simulink model "Simulink_model_pre_alpha"  (R2022b)
settings: Solver=VariableStepAuto  StartTime=0.0  StopTime=10.0  RelTol=1e-3
settings Model: Creator=user  LastModifiedBy=user

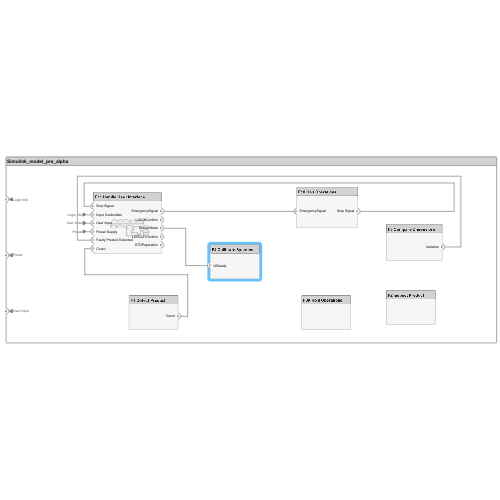
[thumbnail: Simulink's stored preview of the top-level diagram]
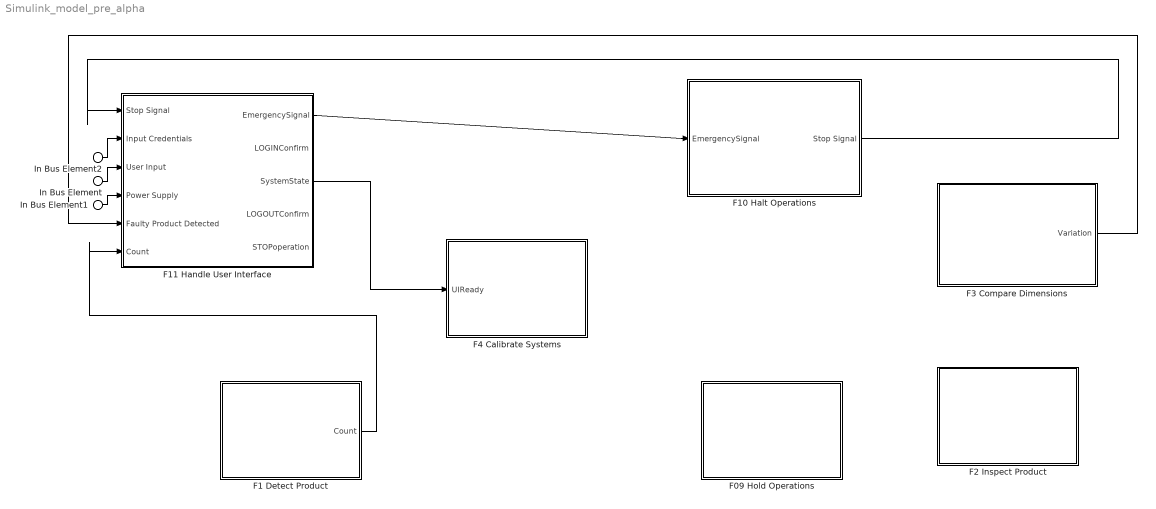
== system Simulink_model_pre_alpha ==
  In Bus Element2 : Inport  PortName=Login info
  In Bus Element1 : Inport  Port=2  PortName=Power
  In Bus Element : Inport  Port=3  PortName=User Input
  F09 Hold Operations : Subsystem
      settings: PortSchema="{\"entries\":[{\"content\":{\"headerSize\":26,\"margin\":15,\"minimumSpacing\":25,\"sides\":[{\"content\":{\"connectorIds\":[]},\"type\":\"ConnectorPlacement.EquallySpacedRectSide\",\"uuid\":\"0eb90d47-70e1-4803-9acf-c665eca2c33b\"},{\"content\":{\"connectorIds\":[],\"side\":\"RIGHT\"},\"type\":\"ConnectorPlacement.EquallySpacedRectSide\",\"uuid\":\"4ca2a7b5-05ae-49c5-bdeb-54cebcfbfa14\"},{\"content\":{\"connectorIds\":[],\"side\":\"TOP\"},\"type\":\"ConnectorPlacement.EquallySpacedRectSide\",\"uuid\":\"0ca0afdf-f9df-4611-9068-250b443486a2\"}]},\"type\":\"ConnectorPlacement.EquallySpacedConnector\",\"uuid\":\"958f48af-2ef9-4d0f-b00d-a4686f354a93\"}],\"packageUris\":[\"http://schema.mathworks.com/mf0/Connector/R2020b\"],\"version\":\"1.0\"}"
  F1 Detect Product : Subsystem
      settings: PortSchema="{\"entries\":[{\"content\":{\"headerSize\":26,\"margin\":15,\"minimumSpacing\":25,\"sides\":[{\"content\":{\"connectorIds\":[]},\"type\":\"ConnectorPlacement.EquallySpacedRectSide\",\"uuid\":\"0eb90d47-70e1-4803-9acf-c665eca2c33b\"},{\"content\":{\"connectorIds\":[\"Out1\"],\"side\":\"RIGHT\"},\"type\":\"ConnectorPlacement.EquallySpacedRectSide\",\"uuid\":\"4ca2a7b5-05ae-49c5-bdeb-54cebcfbfa14\"},{\"content\":{\"connectorIds\":[],\"side\":\"TOP\"},\"type\":\"ConnectorPlacement.EquallySpacedRectSide\",\"uuid\":\"0ca0afdf-f9df-4611-9068-250b443486a2\"}]},\"type\":\"ConnectorPlacement.EquallySpacedConnector\",\"uuid\":\"958f48af-2ef9-4d0f-b00d-a4686f354a93\"}],\"packageUris\":[\"http://schema.mathworks.com/mf0/Connector/R2020b\"],\"version\":\"1.0\"}"
  F10 Halt Operations : Subsystem
      settings: PortSchema="{\"entries\":[{\"content\":{\"headerSize\":26,\"margin\":15,\"minimumSpacing\":25,\"sides\":[{\"content\":{\"connectorIds\":[\"In1\"]},\"type\":\"ConnectorPlacement.EquallySpacedRectSide\",\"uuid\":\"0eb90d47-70e1-4803-9acf-c665eca2c33b\"},{\"content\":{\"connectorIds\":[\"Out1\"],\"side\":\"RIGHT\"},\"type\":\"ConnectorPlacement.EquallySpacedRectSide\",\"uuid\":\"4ca2a7b5-05ae-49c5-bdeb-54cebcfbfa14\"},{\"content\":{\"connectorIds\":[],\"side\":\"TOP\"},\"type\":\"ConnectorPlacement.EquallySpacedRectSide\",\"uuid\":\"0ca0afdf-f9df-4611-9068-250b443486a2\"}]},\"type\":\"ConnectorPlacement.EquallySpacedConnector\",\"uuid\":\"958f48af-2ef9-4d0f-b00d-a4686f354a93\"}],\"packageUris\":[\"http://schema.mathworks.com/mf0/Connector/R2020b\"],\"version\":\"1.0\"}"
  F11 Handle User Interface : Subsystem
      settings: PortSchema="{\"entries\":[{\"content\":{\"headerSize\":26,\"margin\":15,\"minimumSpacing\":25,\"sides\":[{\"content\":{\"connectorIds\":[\"In1\",\"In2\",\"In3\",\"In4\",\"In5\",\"In6\"]},\"type\":\"ConnectorPlacement.EquallySpacedRectSide\",\"uuid\":\"0eb90d47-70e1-4803-9acf-c665eca2c33b\"},{\"content\":{\"connectorIds\":[\"Out1\",\"Out2\",\"Out3\",\"Out4\",\"Out5\"],\"side\":\"RIGHT\"},\"type\":\"ConnectorPlacement.EquallySpacedRectSide\",\"uuid\":\"4ca2a7b5-05ae-49c5-bdeb-54cebcfbfa14\"},{\"content\":{\"connectorIds\":[],\"side\":\"TOP\"},\"type\":\"ConnectorPlacement.EquallySpacedRectSide\",\"uuid\":\"0ca0afdf-f9df-4611-9068-250b443486a2\"}]},\"type\":\"ConnectorPlacement.EquallySpacedConnector\",\"uuid\":\"958f48af-2ef9-4d0f-b00d-a4686f354a93\"}],\"packageUris\":[\"http://schema.mathworks.com/mf0/Connector/R2020b\"],\"version\":\"1.0\"}"
  F2 Inspect Product : Subsystem
      settings: PortSchema="{\"entries\":[{\"content\":{\"headerSize\":26,\"margin\":15,\"minimumSpacing\":25,\"sides\":[{\"content\":{\"connectorIds\":[]},\"type\":\"ConnectorPlacement.EquallySpacedRectSide\",\"uuid\":\"0eb90d47-70e1-4803-9acf-c665eca2c33b\"},{\"content\":{\"connectorIds\":[],\"side\":\"RIGHT\"},\"type\":\"ConnectorPlacement.EquallySpacedRectSide\",\"uuid\":\"4ca2a7b5-05ae-49c5-bdeb-54cebcfbfa14\"},{\"content\":{\"connectorIds\":[],\"side\":\"TOP\"},\"type\":\"ConnectorPlacement.EquallySpacedRectSide\",\"uuid\":\"0ca0afdf-f9df-4611-9068-250b443486a2\"}]},\"type\":\"ConnectorPlacement.EquallySpacedConnector\",\"uuid\":\"958f48af-2ef9-4d0f-b00d-a4686f354a93\"}],\"packageUris\":[\"http://schema.mathworks.com/mf0/Connector/R2020b\"],\"version\":\"1.0\"}"
  F3 Compare Dimensions : Subsystem
      settings: PortSchema="{\"entries\":[{\"content\":{\"headerSize\":26,\"margin\":15,\"minimumSpacing\":25,\"sides\":[{\"content\":{\"connectorIds\":[]},\"type\":\"ConnectorPlacement.EquallySpacedRectSide\",\"uuid\":\"0eb90d47-70e1-4803-9acf-c665eca2c33b\"},{\"content\":{\"connectorIds\":[\"Out1\"],\"side\":\"RIGHT\"},\"type\":\"ConnectorPlacement.EquallySpacedRectSide\",\"uuid\":\"4ca2a7b5-05ae-49c5-bdeb-54cebcfbfa14\"},{\"content\":{\"connectorIds\":[],\"side\":\"TOP\"},\"type\":\"ConnectorPlacement.EquallySpacedRectSide\",\"uuid\":\"0ca0afdf-f9df-4611-9068-250b443486a2\"}]},\"type\":\"ConnectorPlacement.EquallySpacedConnector\",\"uuid\":\"958f48af-2ef9-4d0f-b00d-a4686f354a93\"}],\"packageUris\":[\"http://schema.mathworks.com/mf0/Connector/R2020b\"],\"version\":\"1.0\"}"
  "F4 Calibrate Systems " : Subsystem
      settings: PortSchema="{\"entries\":[{\"content\":{\"headerSize\":26,\"margin\":15,\"minimumSpacing\":25,\"sides\":[{\"content\":{\"connectorIds\":[\"In1\"]},\"type\":\"ConnectorPlacement.EquallySpacedRectSide\",\"uuid\":\"0eb90d47-70e1-4803-9acf-c665eca2c33b\"},{\"content\":{\"connectorIds\":[],\"side\":\"RIGHT\"},\"type\":\"ConnectorPlacement.EquallySpacedRectSide\",\"uuid\":\"4ca2a7b5-05ae-49c5-bdeb-54cebcfbfa14\"},{\"content\":{\"connectorIds\":[],\"side\":\"TOP\"},\"type\":\"ConnectorPlacement.EquallySpacedRectSide\",\"uuid\":\"0ca0afdf-f9df-4611-9068-250b443486a2\"}]},\"type\":\"ConnectorPlacement.EquallySpacedConnector\",\"uuid\":\"958f48af-2ef9-4d0f-b00d-a4686f354a93\"}],\"packageUris\":[\"http://schema.mathworks.com/mf0/Connector/R2020b\"],\"version\":\"1.0\"}"
  wires:
  In Bus Element1/1 -> F11 Handle User Interface/4(Power Supply)
  F10 Halt Operations/1(Stop Signal) -> F11 Handle User Interface/1(Stop Signal)
  In Bus Element/1 -> F11 Handle User Interface/3(User Input)
  In Bus Element2/1 -> F11 Handle User Interface/2(Input Credentials)
  F3 Compare Dimensions/1(Variation) -> F11 Handle User Interface/5(Faulty Product Detected)
  F1 Detect Product/1(Count) -> F11 Handle User Interface/6(Count)
  F11 Handle User Interface/3(SystemState) -> "F4 Calibrate Systems "/1(UIReady)
  F11 Handle User Interface/1(EmergencySignal) -> F10 Halt Operations/1(EmergencySignal)

== system Simulink_model_pre_alpha/F09 Hold Operations ==

== system Simulink_model_pre_alpha/F1 Detect Product ==
  Bus Element Out1 : Outport  PortName=Count

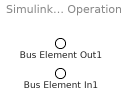
== system Simulink_model_pre_alpha/F10 Halt Operations ==
  Bus Element In1 : Inport  PortName=EmergencySignal
  Bus Element Out1 : Outport  PortName=Stop Signal

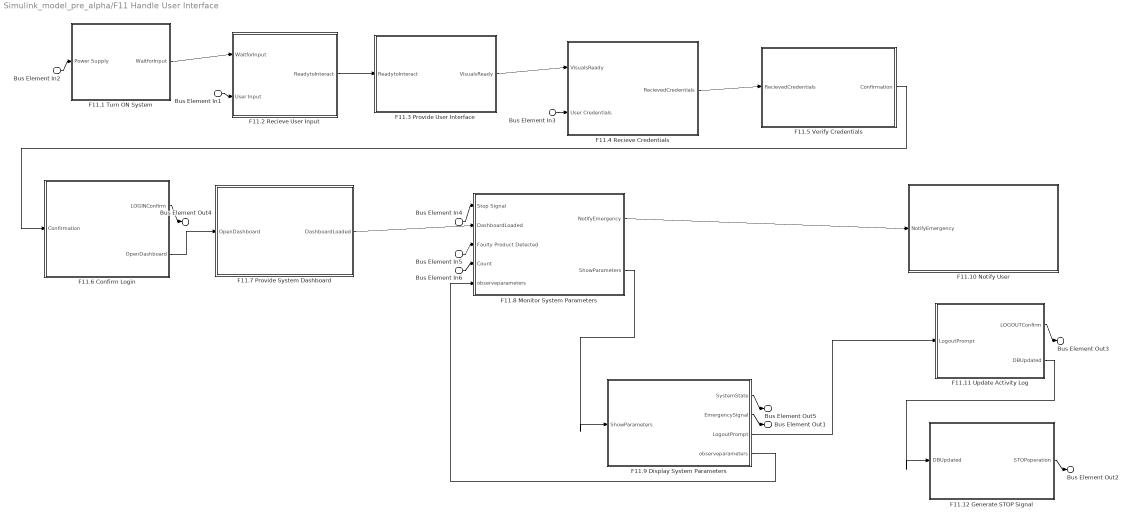
== system Simulink_model_pre_alpha/F11 Handle User Interface ==
  Bus Element In4 : Inport  PortName=Stop Signal
  Bus Element In3 : Inport  Port=2  PortName=Input Credentials
  Bus Element In1 : Inport  Port=3  PortName=User Input
  Bus Element In2 : Inport  Port=4  PortName=Power Supply
  Bus Element In5 : Inport  Port=5  PortName=Faulty Product Detected
  Bus Element In6 : Inport  Port=6  PortName=Count
  F11.1 Turn ON System : Subsystem
      settings: PortSchema="{\"entries\":[{\"content\":{\"headerSize\":26,\"margin\":15,\"minimumSpacing\":25,\"sides\":[{\"content\":{\"connectorIds\":[\"In1\"]},\"type\":\"ConnectorPlacement.EquallySpacedRectSide\",\"uuid\":\"0eb90d47-70e1-4803-9acf-c665eca2c33b\"},{\"content\":{\"connectorIds\":[\"Out1\"],\"side\":\"RIGHT\"},\"type\":\"ConnectorPlacement.EquallySpacedRectSide\",\"uuid\":\"4ca2a7b5-05ae-49c5-bdeb-54cebcfbfa14\"},{\"content\":{\"connectorIds\":[],\"side\":\"TOP\"},\"type\":\"ConnectorPlacement.EquallySpacedRectSide\",\"uuid\":\"0ca0afdf-f9df-4611-9068-250b443486a2\"}]},\"type\":\"ConnectorPlacement.EquallySpacedConnector\",\"uuid\":\"958f48af-2ef9-4d0f-b00d-a4686f354a93\"}],\"packageUris\":[\"http://schema.mathworks.com/mf0/Connector/R2020b\"],\"version\":\"1.0\"}"
  F11.10 Notify User : Subsystem
      settings: PortSchema="{\"entries\":[{\"content\":{\"headerSize\":26,\"margin\":15,\"minimumSpacing\":25,\"sides\":[{\"content\":{\"connectorIds\":[\"In1\"]},\"type\":\"ConnectorPlacement.EquallySpacedRectSide\",\"uuid\":\"0eb90d47-70e1-4803-9acf-c665eca2c33b\"},{\"content\":{\"connectorIds\":[],\"side\":\"RIGHT\"},\"type\":\"ConnectorPlacement.EquallySpacedRectSide\",\"uuid\":\"4ca2a7b5-05ae-49c5-bdeb-54cebcfbfa14\"},{\"content\":{\"connectorIds\":[],\"side\":\"TOP\"},\"type\":\"ConnectorPlacement.EquallySpacedRectSide\",\"uuid\":\"0ca0afdf-f9df-4611-9068-250b443486a2\"}]},\"type\":\"ConnectorPlacement.EquallySpacedConnector\",\"uuid\":\"958f48af-2ef9-4d0f-b00d-a4686f354a93\"}],\"packageUris\":[\"http://schema.mathworks.com/mf0/Connector/R2020b\"],\"version\":\"1.0\"}"
  F11.11 Update Activity Log : Subsystem
      settings: PortSchema="{\"entries\":[{\"content\":{\"headerSize\":26,\"margin\":15,\"minimumSpacing\":25,\"sides\":[{\"content\":{\"connectorIds\":[\"In1\"]},\"type\":\"ConnectorPlacement.EquallySpacedRectSide\",\"uuid\":\"0eb90d47-70e1-4803-9acf-c665eca2c33b\"},{\"content\":{\"connectorIds\":[\"Out1\",\"Out2\"],\"side\":\"RIGHT\"},\"type\":\"ConnectorPlacement.EquallySpacedRectSide\",\"uuid\":\"4ca2a7b5-05ae-49c5-bdeb-54cebcfbfa14\"},{\"content\":{\"connectorIds\":[],\"side\":\"TOP\"},\"type\":\"ConnectorPlacement.EquallySpacedRectSide\",\"uuid\":\"0ca0afdf-f9df-4611-9068-250b443486a2\"}]},\"type\":\"ConnectorPlacement.EquallySpacedConnector\",\"uuid\":\"958f48af-2ef9-4d0f-b00d-a4686f354a93\"}],\"packageUris\":[\"http://schema.mathworks.com/mf0/Connector/R2020b\"],\"version\":\"1.0\"}"
  F11.12 Generate STOP Signal : Subsystem
      settings: PortSchema="{\"entries\":[{\"content\":{\"headerSize\":26,\"margin\":15,\"minimumSpacing\":25,\"sides\":[{\"content\":{\"connectorIds\":[\"In1\"]},\"type\":\"ConnectorPlacement.EquallySpacedRectSide\",\"uuid\":\"0eb90d47-70e1-4803-9acf-c665eca2c33b\"},{\"content\":{\"connectorIds\":[\"Out1\"],\"side\":\"RIGHT\"},\"type\":\"ConnectorPlacement.EquallySpacedRectSide\",\"uuid\":\"4ca2a7b5-05ae-49c5-bdeb-54cebcfbfa14\"},{\"content\":{\"connectorIds\":[],\"side\":\"TOP\"},\"type\":\"ConnectorPlacement.EquallySpacedRectSide\",\"uuid\":\"0ca0afdf-f9df-4611-9068-250b443486a2\"}]},\"type\":\"ConnectorPlacement.EquallySpacedConnector\",\"uuid\":\"958f48af-2ef9-4d0f-b00d-a4686f354a93\"}],\"packageUris\":[\"http://schema.mathworks.com/mf0/Connector/R2020b\"],\"version\":\"1.0\"}"
  F11.2 Recieve User Input : Subsystem
      settings: PortSchema="{\"entries\":[{\"content\":{\"headerSize\":26,\"margin\":15,\"minimumSpacing\":25,\"sides\":[{\"content\":{\"connectorIds\":[\"In1\",\"In2\"]},\"type\":\"ConnectorPlacement.EquallySpacedRectSide\",\"uuid\":\"0eb90d47-70e1-4803-9acf-c665eca2c33b\"},{\"content\":{\"connectorIds\":[\"Out1\"],\"side\":\"RIGHT\"},\"type\":\"ConnectorPlacement.EquallySpacedRectSide\",\"uuid\":\"4ca2a7b5-05ae-49c5-bdeb-54cebcfbfa14\"},{\"content\":{\"connectorIds\":[],\"side\":\"TOP\"},\"type\":\"ConnectorPlacement.EquallySpacedRectSide\",\"uuid\":\"0ca0afdf-f9df-4611-9068-250b443486a2\"}]},\"type\":\"ConnectorPlacement.EquallySpacedConnector\",\"uuid\":\"958f48af-2ef9-4d0f-b00d-a4686f354a93\"}],\"packageUris\":[\"http://schema.mathworks.com/mf0/Connector/R2020b\"],\"version\":\"1.0\"}"
  F11.3 Provide User Interface : Subsystem
      settings: PortSchema="{\"entries\":[{\"content\":{\"headerSize\":26,\"margin\":15,\"minimumSpacing\":25,\"sides\":[{\"content\":{\"connectorIds\":[\"In1\"]},\"type\":\"ConnectorPlacement.EquallySpacedRectSide\",\"uuid\":\"0eb90d47-70e1-4803-9acf-c665eca2c33b\"},{\"content\":{\"connectorIds\":[\"Out1\"],\"side\":\"RIGHT\"},\"type\":\"ConnectorPlacement.EquallySpacedRectSide\",\"uuid\":\"4ca2a7b5-05ae-49c5-bdeb-54cebcfbfa14\"},{\"content\":{\"connectorIds\":[],\"side\":\"TOP\"},\"type\":\"ConnectorPlacement.EquallySpacedRectSide\",\"uuid\":\"0ca0afdf-f9df-4611-9068-250b443486a2\"}]},\"type\":\"ConnectorPlacement.EquallySpacedConnector\",\"uuid\":\"958f48af-2ef9-4d0f-b00d-a4686f354a93\"}],\"packageUris\":[\"http://schema.mathworks.com/mf0/Connector/R2020b\"],\"version\":\"1.0\"}"
  F11.4 Recieve Credentials : Subsystem
      settings: PortSchema="{\"entries\":[{\"content\":{\"headerSize\":26,\"margin\":15,\"minimumSpacing\":25,\"sides\":[{\"content\":{\"connectorIds\":[\"In1\",\"In2\"]},\"type\":\"ConnectorPlacement.EquallySpacedRectSide\",\"uuid\":\"0eb90d47-70e1-4803-9acf-c665eca2c33b\"},{\"content\":{\"connectorIds\":[\"Out1\"],\"side\":\"RIGHT\"},\"type\":\"ConnectorPlacement.EquallySpacedRectSide\",\"uuid\":\"4ca2a7b5-05ae-49c5-bdeb-54cebcfbfa14\"},{\"content\":{\"connectorIds\":[],\"side\":\"TOP\"},\"type\":\"ConnectorPlacement.EquallySpacedRectSide\",\"uuid\":\"0ca0afdf-f9df-4611-9068-250b443486a2\"}]},\"type\":\"ConnectorPlacement.EquallySpacedConnector\",\"uuid\":\"958f48af-2ef9-4d0f-b00d-a4686f354a93\"}],\"packageUris\":[\"http://schema.mathworks.com/mf0/Connector/R2020b\"],\"version\":\"1.0\"}"
  F11.5 Verify Credentials : Subsystem
      settings: PortSchema="{\"entries\":[{\"content\":{\"headerSize\":26,\"margin\":15,\"minimumSpacing\":25,\"sides\":[{\"content\":{\"connectorIds\":[\"In1\"]},\"type\":\"ConnectorPlacement.EquallySpacedRectSide\",\"uuid\":\"0eb90d47-70e1-4803-9acf-c665eca2c33b\"},{\"content\":{\"connectorIds\":[\"Out1\"],\"side\":\"RIGHT\"},\"type\":\"ConnectorPlacement.EquallySpacedRectSide\",\"uuid\":\"4ca2a7b5-05ae-49c5-bdeb-54cebcfbfa14\"},{\"content\":{\"connectorIds\":[],\"side\":\"TOP\"},\"type\":\"ConnectorPlacement.EquallySpacedRectSide\",\"uuid\":\"0ca0afdf-f9df-4611-9068-250b443486a2\"}]},\"type\":\"ConnectorPlacement.EquallySpacedConnector\",\"uuid\":\"958f48af-2ef9-4d0f-b00d-a4686f354a93\"}],\"packageUris\":[\"http://schema.mathworks.com/mf0/Connector/R2020b\"],\"version\":\"1.0\"}"
  F11.6 Confirm Login : Subsystem
      settings: PortSchema="{\"entries\":[{\"content\":{\"headerSize\":26,\"margin\":15,\"minimumSpacing\":25,\"sides\":[{\"content\":{\"connectorIds\":[\"In1\"]},\"type\":\"ConnectorPlacement.EquallySpacedRectSide\",\"uuid\":\"0eb90d47-70e1-4803-9acf-c665eca2c33b\"},{\"content\":{\"connectorIds\":[\"Out1\",\"Out2\"],\"side\":\"RIGHT\"},\"type\":\"ConnectorPlacement.EquallySpacedRectSide\",\"uuid\":\"4ca2a7b5-05ae-49c5-bdeb-54cebcfbfa14\"},{\"content\":{\"connectorIds\":[],\"side\":\"TOP\"},\"type\":\"ConnectorPlacement.EquallySpacedRectSide\",\"uuid\":\"0ca0afdf-f9df-4611-9068-250b443486a2\"}]},\"type\":\"ConnectorPlacement.EquallySpacedConnector\",\"uuid\":\"958f48af-2ef9-4d0f-b00d-a4686f354a93\"}],\"packageUris\":[\"http://schema.mathworks.com/mf0/Connector/R2020b\"],\"version\":\"1.0\"}"
  F11.7 Provide System Dashboard : Subsystem
      settings: PortSchema="{\"entries\":[{\"content\":{\"headerSize\":26,\"margin\":15,\"minimumSpacing\":25,\"sides\":[{\"content\":{\"connectorIds\":[\"In1\"]},\"type\":\"ConnectorPlacement.EquallySpacedRectSide\",\"uuid\":\"0eb90d47-70e1-4803-9acf-c665eca2c33b\"},{\"content\":{\"connectorIds\":[\"Out1\"],\"side\":\"RIGHT\"},\"type\":\"ConnectorPlacement.EquallySpacedRectSide\",\"uuid\":\"4ca2a7b5-05ae-49c5-bdeb-54cebcfbfa14\"},{\"content\":{\"connectorIds\":[],\"side\":\"TOP\"},\"type\":\"ConnectorPlacement.EquallySpacedRectSide\",\"uuid\":\"0ca0afdf-f9df-4611-9068-250b443486a2\"}]},\"type\":\"ConnectorPlacement.EquallySpacedConnector\",\"uuid\":\"958f48af-2ef9-4d0f-b00d-a4686f354a93\"}],\"packageUris\":[\"http://schema.mathworks.com/mf0/Connector/R2020b\"],\"version\":\"1.0\"}"
  F11.8 Monitor System Parameters : Subsystem
      settings: PortSchema="{\"entries\":[{\"content\":{\"headerSize\":26,\"margin\":15,\"minimumSpacing\":25,\"sides\":[{\"content\":{\"connectorIds\":[\"In1\",\"In2\",\"In3\",\"In5\",\"In4\"]},\"type\":\"ConnectorPlacement.EquallySpacedRectSide\",\"uuid\":\"0eb90d47-70e1-4803-9acf-c665eca2c33b\"},{\"content\":{\"connectorIds\":[\"Out1\",\"Out2\"],\"side\":\"RIGHT\"},\"type\":\"ConnectorPlacement.EquallySpacedRectSide\",\"uuid\":\"4ca2a7b5-05ae-49c5-bdeb-54cebcfbfa14\"},{\"content\":{\"connectorIds\":[],\"side\":\"TOP\"},\"type\":\"ConnectorPlacement.EquallySpacedRectSide\",\"uuid\":\"0ca0afdf-f9df-4611-9068-250b443486a2\"}]},\"type\":\"ConnectorPlacement.EquallySpacedConnector\",\"uuid\":\"958f48af-2ef9-4d0f-b00d-a4686f354a93\"}],\"packageUris\":[\"http://schema.mathworks.com/mf0/Connector/R2020b\"],\"version\":\"1.0\"}"
  F11.9 Display System Parameters : Subsystem
      settings: PortSchema="{\"entries\":[{\"content\":{\"headerSize\":26,\"margin\":15,\"minimumSpacing\":25,\"sides\":[{\"content\":{\"connectorIds\":[\"In1\"]},\"type\":\"ConnectorPlacement.EquallySpacedRectSide\",\"uuid\":\"0eb90d47-70e1-4803-9acf-c665eca2c33b\"},{\"content\":{\"connectorIds\":[\"Out1\",\"Out2\",\"Out3\",\"Out4\"],\"side\":\"RIGHT\"},\"type\":\"ConnectorPlacement.EquallySpacedRectSide\",\"uuid\":\"4ca2a7b5-05ae-49c5-bdeb-54cebcfbfa14\"},{\"content\":{\"connectorIds\":[],\"side\":\"TOP\"},\"type\":\"ConnectorPlacement.EquallySpacedRectSide\",\"uuid\":\"0ca0afdf-f9df-4611-9068-250b443486a2\"}]},\"type\":\"ConnectorPlacement.EquallySpacedConnector\",\"uuid\":\"958f48af-2ef9-4d0f-b00d-a4686f354a93\"}],\"packageUris\":[\"http://schema.mathworks.com/mf0/Connector/R2020b\"],\"version\":\"1.0\"}"
  Bus Element Out1 : Outport  PortName=EmergencySignal
  Bus Element Out4 : Outport  Port=2  PortName=LOGINConfirm
  Bus Element Out5 : Outport  Port=3  PortName=SystemState
  Bus Element Out3 : Outport  Port=4  PortName=LOGOUTConfirm
  Bus Element Out2 : Outport  Port=5  PortName=STOPoperation
  wires:
  Bus Element In2/1 -> F11.1 Turn ON System/1(Power Supply)
  F11.1 Turn ON System/1(WaitforInput) -> F11.2 Recieve User Input/1(WaitforInput)
  Bus Element In1/1 -> F11.2 Recieve User Input/2(User Input)
  F11.2 Recieve User Input/1(ReadytoInteract) -> F11.3 Provide User Interface/1(ReadytoInteract)
  F11.3 Provide User Interface/1(VisualsReady) -> F11.4 Recieve Credentials/1(VisualsReady)
  Bus Element In3/1 -> F11.4 Recieve Credentials/2(User Credentials)
  F11.4 Recieve Credentials/1(RecievedCredentials) -> F11.5 Verify Credentials/1(RecievedCredentials)
  F11.5 Verify Credentials/1(Confirmation) -> F11.6 Confirm Login/1(Confirmation)
  F11.6 Confirm Login/2(OpenDashboard) -> F11.7 Provide System Dashboard/1(OpenDashboard)
  F11.7 Provide System Dashboard/1(DashboardLoaded) -> F11.8 Monitor System Parameters/2(DashboardLoaded)
  Bus Element In4/1 -> F11.8 Monitor System Parameters/1(Stop Signal)
  Bus Element In5/1 -> F11.8 Monitor System Parameters/3(Faulty Product Detected)
  Bus Element In6/1 -> F11.8 Monitor System Parameters/5(Count)
  F11.8 Monitor System Parameters/2(ShowParameters) -> F11.9 Display System Parameters/1(ShowParameters)
  F11.8 Monitor System Parameters/1(NotifyEmergency) -> F11.10 Notify User/1(NotifyEmergency)
  F11.9 Display System Parameters/2(EmergencySignal) -> Bus Element Out1/1
  F11.9 Display System Parameters/4(observeparameters) -> F11.8 Monitor System Parameters/4(observeparameters)
  F11.9 Display System Parameters/3(LogoutPrompt) -> F11.11 Update Activity Log/1(LogoutPrompt)
  F11.12 Generate STOP Signal/1(STOPoperation) -> Bus Element Out2/1
  F11.11 Update Activity Log/1(LOGOUTConfirm) -> Bus Element Out3/1
  F11.6 Confirm Login/1(LOGINConfirm) -> Bus Element Out4/1
  F11.9 Display System Parameters/1(SystemState) -> Bus Element Out5/1
  F11.11 Update Activity Log/2(DBUpdated) -> F11.12 Generate STOP Signal/1(DBUpdated)

== system Simulink_model_pre_alpha/F2 Inspect Product ==

== system Simulink_model_pre_alpha/F3 Compare Dimensions ==
  Bus Element Out1 : Outport  PortName=Variation

== system Simulink_model_pre_alpha/F4 Calibrate Systems  ==
  Bus Element In1 : Inport  PortName=UIReady

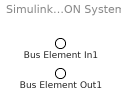
== system Simulink_model_pre_alpha/F11 Handle User Interface/F11.1 Turn ON System ==
  Bus Element In1 : Inport  PortName=Power Supply
  Bus Element Out1 : Outport  PortName=WaitforInput

== system Simulink_model_pre_alpha/F11 Handle User Interface/F11.10 Notify User ==
  Bus Element In1 : Inport  PortName=NotifyEmergency

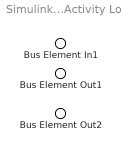
== system Simulink_model_pre_alpha/F11 Handle User Interface/F11.11 Update Activity Log ==
  Bus Element In1 : Inport  PortName=LogoutPrompt
  Bus Element Out1 : Outport  PortName=LOGOUTConfirm
  Bus Element Out2 : Outport  Port=2  PortName=DBUpdated

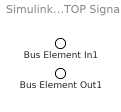
== system Simulink_model_pre_alpha/F11 Handle User Interface/F11.12 Generate STOP Signal ==
  Bus Element In1 : Inport  PortName=DBUpdated
  Bus Element Out1 : Outport  PortName=STOPoperation

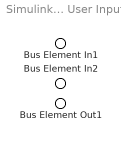
== system Simulink_model_pre_alpha/F11 Handle User Interface/F11.2 Recieve User Input ==
  Bus Element In1 : Inport  PortName=WaitforInput
  Bus Element In2 : Inport  Port=2  PortName=User Input
  Bus Element Out1 : Outport  PortName=ReadytoInteract

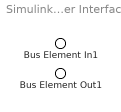
== system Simulink_model_pre_alpha/F11 Handle User Interface/F11.3 Provide User Interface ==
  Bus Element In1 : Inport  PortName=ReadytoInteract
  Bus Element Out1 : Outport  PortName=VisualsReady

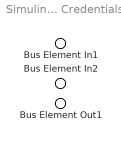
== system Simulink_model_pre_alpha/F11 Handle User Interface/F11.4 Recieve Credentials ==
  Bus Element In1 : Inport  PortName=VisualsReady
  Bus Element In2 : Inport  Port=2  PortName=User Credentials
  Bus Element Out1 : Outport  PortName=RecievedCredentials

== system Simulink_model_pre_alpha/F11 Handle User Interface/F11.5 Verify Credentials ==
  Bus Element In1 : Inport  PortName=RecievedCredentials
  Bus Element Out1 : Outport  PortName=Confirmation

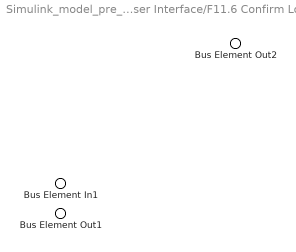
== system Simulink_model_pre_alpha/F11 Handle User Interface/F11.6 Confirm Login ==
  Bus Element In1 : Inport  PortName=Confirmation
  Bus Element Out2 : Outport  PortName=LOGINConfirm
  Bus Element Out1 : Outport  Port=2  PortName=OpenDashboard

== system Simulink_model_pre_alpha/F11 Handle User Interface/F11.7 Provide System Dashboard ==
  Bus Element In1 : Inport  PortName=OpenDashboard
  Bus Element Out1 : Outport  PortName=DashboardLoaded

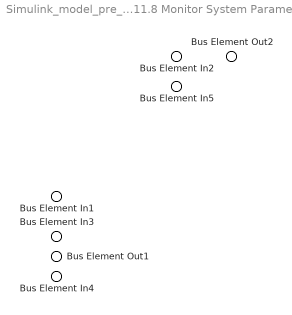
== system Simulink_model_pre_alpha/F11 Handle User Interface/F11.8 Monitor System Parameters ==
  Bus Element In2 : Inport  PortName=Stop Signal
  Bus Element In1 : Inport  Port=2  PortName=DashboardLoaded
  Bus Element In3 : Inport  Port=3  PortName=Faulty Product Detected
  Bus Element In5 : Inport  Port=4  PortName=observeparameters
  Bus Element In4 : Inport  Port=5  PortName=Count
  Bus Element Out2 : Outport  PortName=NotifyEmergency
  Bus Element Out1 : Outport  Port=2  PortName=ShowParameters

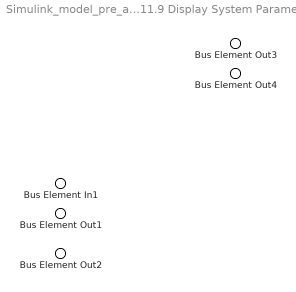
== system Simulink_model_pre_alpha/F11 Handle User Interface/F11.9 Display System Parameters ==
  Bus Element In1 : Inport  PortName=ShowParameters
  Bus Element Out4 : Outport  PortName=SystemState
  Bus Element Out1 : Outport  Port=2  PortName=EmergencySignal
  Bus Element Out3 : Outport  Port=3  PortName=LogoutPrompt
  Bus Element Out2 : Outport  Port=4  PortName=observeparameters
